simulink model "spinEchoNetwork"  (R2014a)
settings: Solver=FixedStepDiscrete  StartTime=1  StopTime=1  FixedStep=1  RelTol=1e-3
libraries: opticalComponentLibrary x7
settings Model: Creator=Nithya Menon  LastModifiedBy=Alexander
settings DebuggingCC: UnderspecifiedInitializationDetection=Classic  StateNameClashWarn=warning

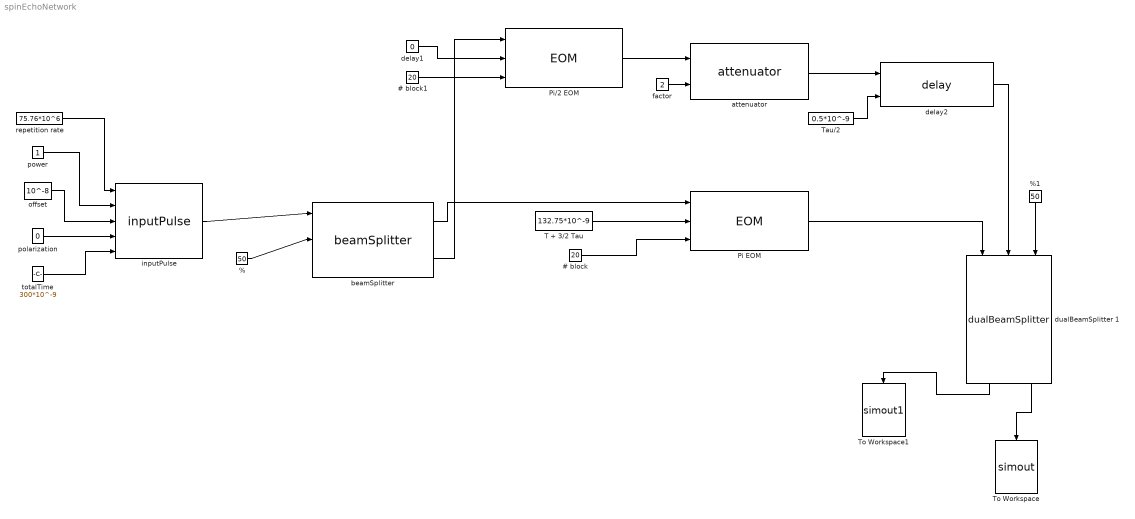
== system spinEchoNetwork ==
  # block : Constant  Value=20
  # block1 : Constant  Value=20
  % : Constant  Value=50
  %1 : Constant  Value=50
  Pi EOM : opticalComponentLibrary/EOM
  Pi/2 EOM : opticalComponentLibrary/EOM
  T + 3/2 Tau : Constant  Value=132.75*10^-9
  Tau/2 : Constant  Value=0.5*10^-9
  To Workspace : ToWorkspace  VariableName=simout  SaveFormat=Structure  SampleTime=-1
  To Workspace1 : ToWorkspace  VariableName=simout1  SaveFormat=Structure  SampleTime=-1
  attenuator : opticalComponentLibrary/attenuator
  beamSplitter : opticalComponentLibrary/beamSplitter
  delay1 : Constant  Value=0
  delay2 : opticalComponentLibrary/delay
  dualBeamSplitter 1 : opticalComponentLibrary/dualBeamSplitter 
  factor : Constant  Value=2
  inputPulse : opticalComponentLibrary/inputPulse
  offset : Constant  Value=10^-8
  polarization : Constant  Value=0
  power : Constant
  repetition rate : Constant  Value=75.76*10^6
  totalTime : Constant  Value=300*10^-9
  wires:
  polarization/1 -> inputPulse/4
  offset/1 -> inputPulse/3
  power/1 -> inputPulse/2
  repetition rate/1 -> inputPulse/1
  %/1 -> beamSplitter/2
  beamSplitter/1 -> Pi EOM/1
  T + 3/2 Tau/1 -> Pi EOM/2
  # block/1 -> Pi EOM/3
  Pi EOM/1 -> dualBeamSplitter 1/1
  beamSplitter/2 -> Pi/2 EOM/1
  delay1/1 -> Pi/2 EOM/2
  # block1/1 -> Pi/2 EOM/3
  Pi/2 EOM/1 -> attenuator/1
  factor/1 -> attenuator/2
  attenuator/1 -> delay2/1
  delay2/1 -> dualBeamSplitter 1/2
  Tau/2/1 -> delay2/2
  inputPulse/1 -> beamSplitter/1
  %1/1 -> dualBeamSplitter 1/3
  dualBeamSplitter 1/2 -> To Workspace/1
  dualBeamSplitter 1/1 -> To Workspace1/1
  totalTime/1 -> inputPulse/5
